simulink model "sdpm_vector_velocity"  (Simulink 9.0)
settings: Solver=ode45  StartTime=0.0  StopTime=5  RelTol=1e-7  AbsTol=1e-7  EnableMultiTasking=on
values from neighbouring files (symbols this model uses):
  c = 5    [index.m]
  iff = 10*0.71    (= 7.1)    [index.m]
  J = 0.00001    (= 1e-05)    [index.m]
  J2 = 0.000215    [index.m]
  ki1 = 20000    [index.m]
  kii = ki*ki/4    (= 109202500)    [index.m]
  km = 3*(Lm*iff*pn)/2    (= 0.19809)    [index.m]
  kw = 0.04    [index.m]
  L = 0.008    [index.m]
  Lm = 0.0062    [index.m]
  nu = 0.00007/2    (= 3.5e-05)    [index.m]
  nu2 = nu    (= 3.5e-05)    [index.m]
  nu3 = 0.01    [index.m]
  pn = 3    [index.m]
  R = 7.2    [index.m]
  tau = 1/wo    [index.m]
settings Model: Creator=Alex  LastModifiedBy=Alexander
settings DataIOCC: LimitDataPoints=on  SignalLoggingSaveFormat=ModelDataLogs
settings OptimizationCC: ExpressionDepthLimit=2147483647
settings DebuggingCC: SolverPrmCheckMsg=warning  FcnCallInpInsideContextMsg=warning  StateNameClashWarn=warning
settings GRTTargetCC: GeneratePreprocessorConditionals=Disable all  CombineOutputUpdateFcns=off  GRTInterface=on

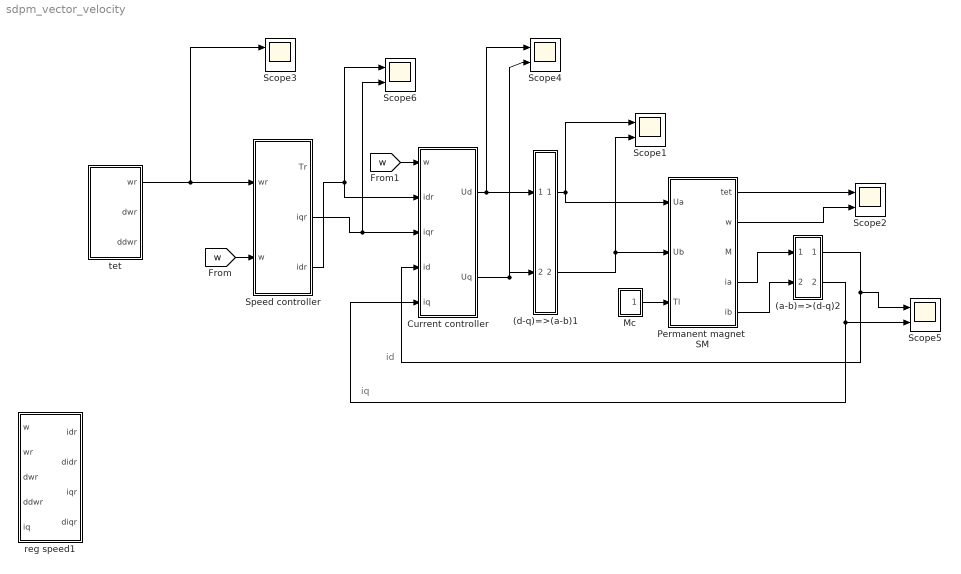
== system sdpm_vector_velocity ==
  note: id
  note: iq
  (a-b)=>(d-q)2 : Subsystem
  (d-q)=>(a-b)1 : Subsystem
  Current controller : Subsystem
  Mc : Subsystem  mask{te=1, td=1.5, Mc=0}
      mask prompts: te "Enable time"; td "Disable time"
  Permanent magnet  SM : Subsystem
  Scope{1..6} (6 alike) : Scope  NumInputPorts=2
  Speed controller : Subsystem
  reg speed1 : Subsystem  mask{kw=100, J=0.003, km=0.636, ktet=0}
      mask init:
      | kwi=(kw*kw)/2
  tet : Subsystem  mask{wrmax=1000, ta=0.5, ka=0.2, tcon=1, tex=0.5}
      mask prompts: wrmax "Final speed value"; ta "Ramp time"; ka "Coef. smooth"; tcon "Const speed time"; tex "Excitation time"
  wires:
  Mc/1(Mc) -> Permanent magnet  SM/3(Tl)
  tet/1(wr) -> Scope3/1, Speed controller/1(wr)
  Current controller/2(Uq) -> (d-q)=>(a-b)1/2("q "), Scope4/2
  (d-q)=>(a-b)1/2(b) -> Scope1/2, Permanent magnet  SM/2(Ub)
  (d-q)=>(a-b)1/1(a) -> Scope1/1, Permanent magnet  SM/1(Ua)
  (a-b)=>(d-q)2/2(q) -> Scope5/2, Current controller/5(iq)
  Speed controller/2("iqr  ") -> Scope6/2, Current controller/3(iqr)
  Current controller/1(Ud) -> Scope4/1, (d-q)=>(a-b)1/1(d)
  (a-b)=>(d-q)2/1(d) -> Scope5/1, Current controller/4(id)
  Speed controller/3(idr) -> Scope6/1, Current controller/2(idr)
  [w] -> Speed controller/2("w ")
  [w] -> Current controller/1(w)
  Permanent magnet  SM/1(tet) -> Scope2/1
  Permanent magnet  SM/2(w) -> Scope2/2
  Permanent magnet  SM/4(ia) -> (a-b)=>(d-q)2/1(a)
  Permanent magnet  SM/5(ib) -> (a-b)=>(d-q)2/2("b ")

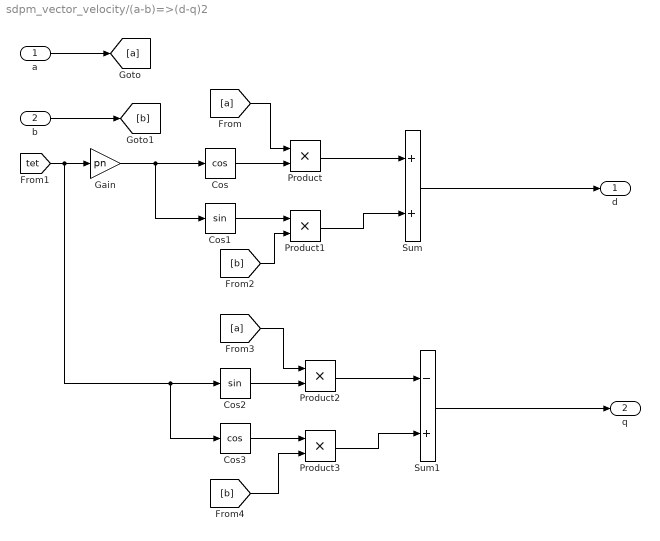
== system sdpm_vector_velocity/(a-b)=>(d-q)2 ==
  a : Inport
  "b " : Inport  Port=2
  Cos : Trigonometry  Operator=cos
  Cos1 : Trigonometry
  Cos2 : Trigonometry
  Cos3 : Trigonometry  Operator=cos
  Gain : Gain  Gain=pn
  Product{,1..3} (4 alike) : Product
  Sum : Sum
  Sum1 : Sum  Inputs=-+
  d : Outport
  q : Outport  Port=2
  wires:
  [b] -> Product1/2
  [b] -> Product3/2
  a/1 -> [a]
  [a] -> Product/1
  Sum/1 -> d/1
  [a] -> Product2/1
  Sum1/1 -> q/1
  Cos3/1 -> Product3/1
  Product3/1 -> Sum1/2
  Product/1 -> Sum/1
  Product2/1 -> Sum1/1
  Gain/1 -> Cos1/1, Cos/1
  Product1/1 -> Sum/2
  Cos1/1 -> Product1/1
  "b "/1 -> [b]
  Cos/1 -> Product/2
  [tet] -> Cos3/1, Cos2/1, Gain/1
  Cos2/1 -> Product2/2

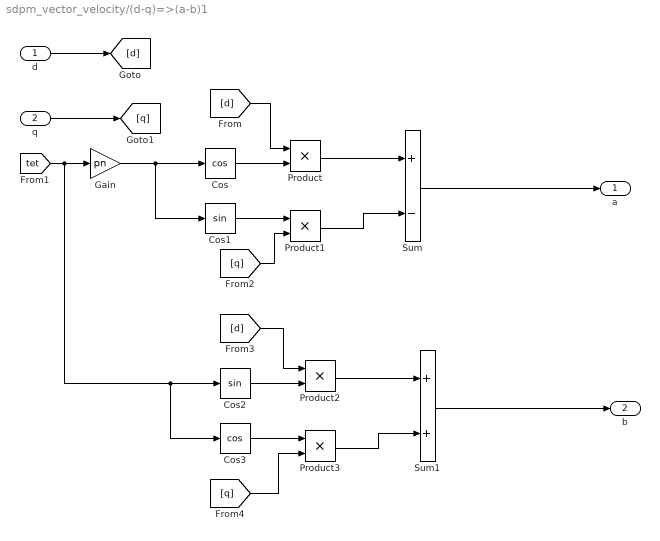
== system sdpm_vector_velocity/(d-q)=>(a-b)1 ==
  d : Inport
  "q " : Inport  Port=2
  Cos : Trigonometry  Operator=cos
  Cos1 : Trigonometry
  Cos2 : Trigonometry
  Cos3 : Trigonometry  Operator=cos
  Gain : Gain  Gain=pn
  Product{,1..3} (4 alike) : Product
  Sum : Sum  Inputs=+-
  Sum1 : Sum
  a : Outport
  b : Outport  Port=2
  wires:
  Gain/1 -> Cos1/1, Cos/1
  Cos/1 -> Product/2
  Product/1 -> Sum/1
  Cos1/1 -> Product1/1
  Product1/1 -> Sum/2
  Sum/1 -> a/1
  Product2/1 -> Sum1/1
  Cos2/1 -> Product2/2
  Sum1/1 -> b/1
  [tet] -> Cos3/1, Cos2/1, Gain/1
  Product3/1 -> Sum1/2
  Cos3/1 -> Product3/1
  d/1 -> [d]
  "q "/1 -> [q]
  [d] -> Product/1
  [q] -> Product1/2
  [d] -> Product2/1
  [q] -> Product3/2

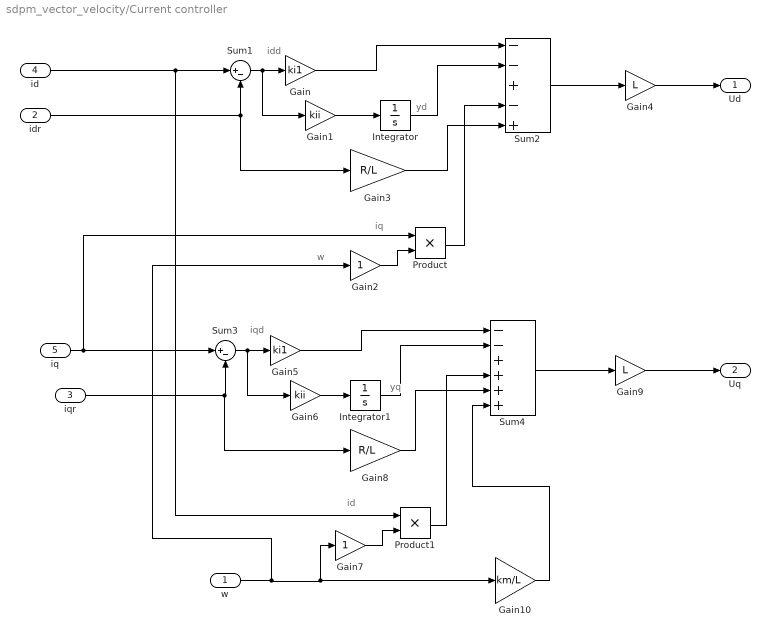
== system sdpm_vector_velocity/Current controller ==
  note: yq
  note: iqd
  note: yd
  note: idd
  note: w
  note: iq
  note: id
  w : Inport
  idr : Inport  Port=2
  iqr : Inport  Port=3
  id : Inport  Port=4
  iq : Inport  Port=5
  Gain : Gain  Gain=ki1
  Gain1 : Gain  Gain=kii
  Gain10 : Gain  Gain=km/L
  Gain2 : Gain
  Gain3 : Gain  Gain=R/L
  Gain4 : Gain  Gain=L
  Gain5 : Gain  Gain=ki1
  Gain6 : Gain  Gain=kii
  Gain7 : Gain
  Gain8 : Gain  Gain=R/L
  Gain9 : Gain  Gain=L
  Integrator : Integrator
  Integrator1 : Integrator
  Product : Product
  Product1 : Product
  Sum1 : Sum  Inputs=|+-
  Sum2 : Sum  Inputs=--+-+
  Sum3 : Sum  Inputs=|+-
  Sum4 : Sum  Inputs=--++++
  Ud : Outport
  Uq : Outport  Port=2
  wires:
  Product/1 -> Sum2/4
  Sum2/1 -> Gain4/1
  w/1 -> Gain7/1, Gain10/1, Gain2/1
  Integrator1/1 -> Sum4/2
  Gain7/1 -> Product1/2
  Gain8/1 -> Sum4/5
  Sum4/1 -> Gain9/1
  Gain9/1 -> Uq/1
  Product1/1 -> Sum4/4
  Gain6/1 -> Integrator1/1
  Sum3/1 -> Gain5/1, Gain6/1
  iqr/1 -> Sum3/2, Gain8/1
  Gain5/1 -> Sum4/1
  Gain4/1 -> Ud/1
  idr/1 -> Sum1/2, Gain3/1
  Sum1/1 -> Gain/1, Gain1/1
  id/1 -> Sum1/1, Product1/1
  iq/1 -> Product/1, Sum3/1
  Gain2/1 -> Product/2
  Gain/1 -> Sum2/1
  Gain10/1 -> Sum4/6
  Integrator/1 -> Sum2/2
  Gain3/1 -> Sum2/5
  Gain1/1 -> Integrator/1

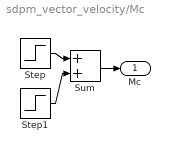
== system sdpm_vector_velocity/Mc ==
  Step : Step  Time=te  After=Mc
  Step1 : Step  Time=td  After=-Mc
  Sum : Sum  SaturateOnIntegerOverflow=on  InputSameDT=on  OutDataTypeStr=Inherit: Same as first input
  Mc : Outport
  wires:
  Step/1 -> Sum/1
  Step1/1 -> Sum/2
  Sum/1 -> Mc/1

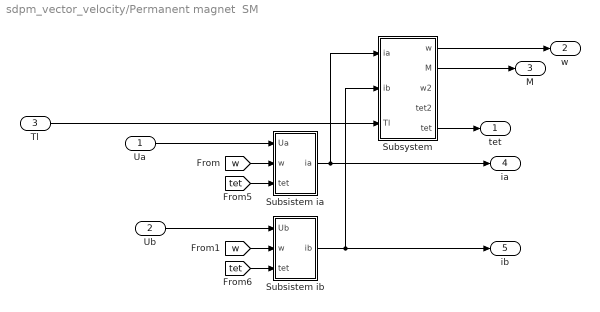
== system sdpm_vector_velocity/Permanent magnet  SM ==
  Ua : Inport
  Ub : Inport  Port=2
  Tl : Inport  Port=3
  Subsistem ia : Subsystem
  Subsistem ib : Subsystem
  Subsystem : Subsystem
  tet : Outport
  w : Outport  Port=2
  M : Outport  Port=3
  ia : Outport  Port=4
  ib : Outport  Port=5
  wires:
  Ua/1 -> Subsistem ia/1(Ua)
  Subsistem ia/1(ia) -> ia/1, Subsystem/1(ia)
  Ub/1 -> Subsistem ib/1(Ub)
  Subsistem ib/1(ib) -> ib/1, Subsystem/2(ib)
  Subsystem/2(M) -> M/1
  Tl/1 -> Subsystem/3("Tl ")
  Subsystem/1(w) -> w/1
  [w] -> Subsistem ia/2(w)
  [w] -> Subsistem ib/2(w)
  [tet] -> Subsistem ia/3(tet)
  [tet] -> Subsistem ib/3(tet)
  Subsystem/5(tet) -> tet/1

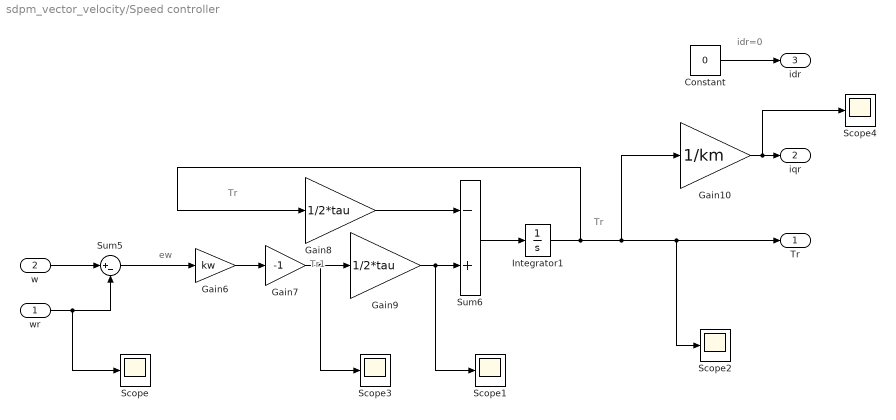
== system sdpm_vector_velocity/Speed controller ==
  note: idr=0
  note: Tr1
  note: ew
  note: Tr
  note: Tr
  wr : Inport
  "w " : Inport  Port=2
  Constant : Constant  Value=0
  Gain10 : Gain  Gain=1/km
  Gain6 : Gain  Gain=kw
  Gain7 : Gain  Gain=-1
  Gain8 : Gain  Gain=1/2*tau
  Gain9 : Gain  Gain=1/2*tau
  Integrator1 : Integrator
  Scope{,1..4} (5 alike) : Scope
  Sum5 : Sum  Inputs=|+-
  Sum6 : Sum  Inputs=-+
  Tr : Outport
  "iqr  " : Outport  Port=2
  idr : Outport  Port=3
  wires:
  wr/1 -> Scope/1, Sum5/2
  "w "/1 -> Sum5/1
  Sum5/1 -> Gain6/1
  Gain6/1 -> Gain7/1
  Gain7/1 -> Scope3/1, Gain9/1
  Integrator1/1 -> Gain8/1, Gain10/1, Scope2/1, Tr/1
  Sum6/1 -> Integrator1/1
  Gain9/1 -> Scope1/1, Sum6/2
  Gain8/1 -> Sum6/1
  Gain10/1 -> Scope4/1, "iqr  "/1
  Constant/1 -> idr/1

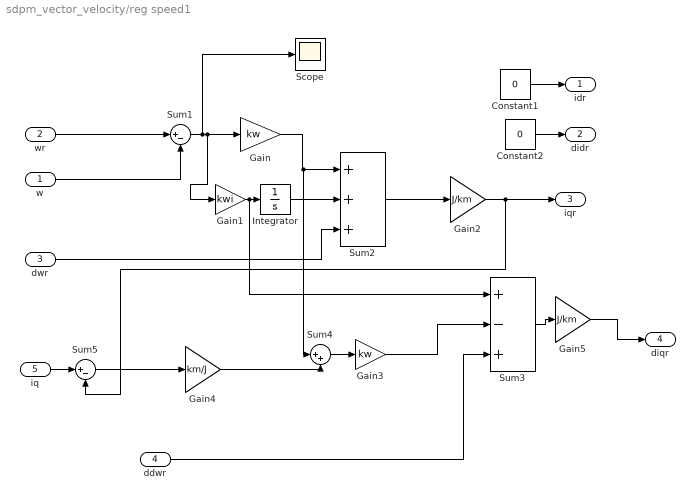
== system sdpm_vector_velocity/reg speed1 ==
  w : Inport
  wr : Inport  Port=2
  dwr : Inport  Port=3
  ddwr : Inport  Port=4
  iq : Inport  Port=5
  Constant1 : Constant  Value=0
  Constant2 : Constant  Value=0
  Gain : Gain  Gain=kw
  Gain1 : Gain  Gain=kwi
  Gain2 : Gain  Gain=J/km
  Gain3 : Gain  Gain=kw
  Gain4 : Gain  Gain=km/J
  Gain5 : Gain  Gain=J/km
  Integrator : Integrator
  Scope : Scope
  Sum1 : Sum  Inputs=|+-
  Sum2 : Sum  Inputs=+++
  Sum3 : Sum  Inputs=+-+
  Sum4 : Sum  Inputs=|++
  Sum5 : Sum  Inputs=|+-
  idr : Outport
  didr : Outport  Port=2
  iqr : Outport  Port=3
  diqr : Outport  Port=4
  wires:
  dwr/1 -> Sum2/3
  Gain5/1 -> diqr/1
  Sum3/1 -> Gain5/1
  ddwr/1 -> Sum3/3
  Gain3/1 -> Sum3/2
  Sum5/1 -> Gain4/1
  Gain4/1 -> Sum4/2
  Sum4/1 -> Gain3/1
  Integrator/1 -> Sum2/2
  Sum2/1 -> Gain2/1
  Gain2/1 -> iqr/1, Sum5/2
  w/1 -> Sum1/2
  wr/1 -> Sum1/1
  Gain1/1 -> Integrator/1, Sum3/1
  Sum1/1 -> Gain/1, Gain1/1, Scope/1
  Gain/1 -> Sum2/1, Sum4/1
  iq/1 -> Sum5/1
  Constant1/1 -> idr/1
  Constant2/1 -> didr/1

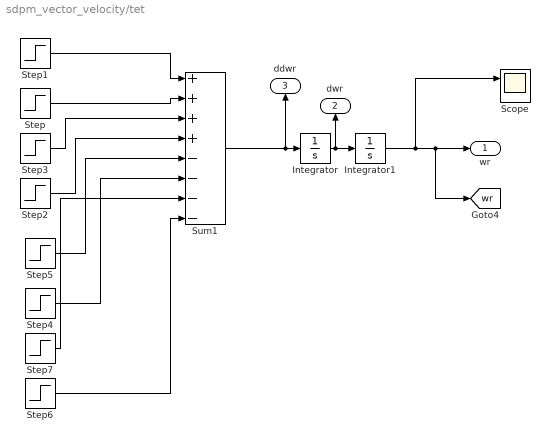
== system sdpm_vector_velocity/tet ==
  Integrator : Integrator
  Integrator1 : Integrator
  Scope : Scope  NumInputPorts=2
  Step : Step  Time=tex+ta*ka  After=-wrmax/(ka*ta*ka*ta+ka*ta*(ta-2*ka*ta))
  Step1 : Step  Time=tex  After=wrmax/(ka*ta*ka*ta+ka*ta*(ta-2*ka*ta))
  Step2 : Step  Time=tex+ta  After=wrmax/(ka*ta*ka*ta+ka*ta*(ta-2*ka*ta))
  Step3 : Step  Time=tex+ta*ka+(ta-2*ta*ka)  After=-wrmax/(ka*ta*ka*ta+ka*ta*(ta-2*ka*ta))
  Step4 : Step  Time=tex+ta+tcon+ta*ka  After=-wrmax/(ka*ta*ka*ta+ka*ta*(ta-2*ka*ta))
  Step5 : Step  Time=tex+ta+tcon  After=wrmax/(ka*ta*ka*ta+ka*ta*(ta-2*ka*ta))
  Step6 : Step  Time=tex+ta+tcon+ta  After=wrmax/(ka*ta*ka*ta+ka*ta*(ta-2*ka*ta))
  Step7 : Step  Time=tex+ta+tcon+ta*ka+(ta-2*ta*ka)  After=-wrmax/(ka*ta*ka*ta+ka*ta*(ta-2*ka*ta))
  Sum1 : Sum  Inputs=++++----  SaturateOnIntegerOverflow=on  InputSameDT=on  OutDataTypeStr=Inherit: Same as first input
  wr : Outport  InitialOutput=0
  dwr : Outport  Port=2  InitialOutput=0
  ddwr : Outport  Port=3  InitialOutput=0
  tag scope: wr=global
  wires:
  Step6/1 -> Sum1/8
  Step7/1 -> Sum1/7
  Step4/1 -> Sum1/6
  Integrator/1 -> dwr/1, Integrator1/1
  Sum1/1 -> Integrator/1, ddwr/1
  Integrator1/1 -> wr/1, [wr], Scope/1
  Step5/1 -> Sum1/5
  Step2/1 -> Sum1/4
  Step3/1 -> Sum1/3
  Step/1 -> Sum1/2
  Step1/1 -> Sum1/1

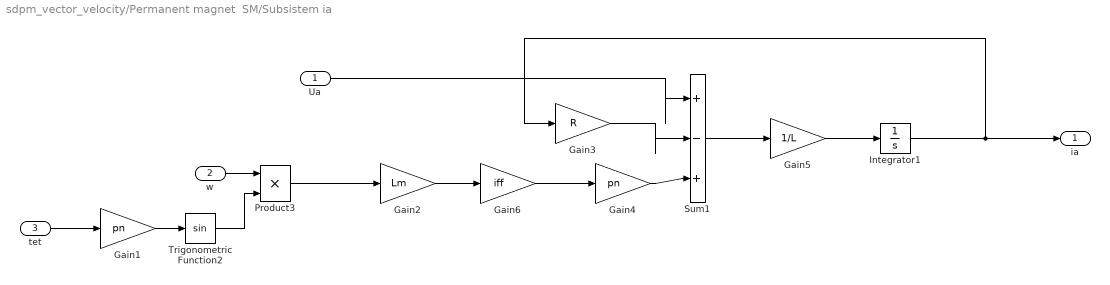
== system sdpm_vector_velocity/Permanent magnet  SM/Subsistem ia ==
  Ua : Inport
  w : Inport  Port=2
  tet : Inport  Port=3
  Gain1 : Gain  Gain=pn  SaturateOnIntegerOverflow=on  OutDataTypeStr=Inherit: Same as input  ParamDataTypeStr=Inherit: Same as input
  Gain2 : Gain  Gain=Lm  SaturateOnIntegerOverflow=on  OutDataTypeStr=Inherit: Same as input  ParamDataTypeStr=Inherit: Same as input
  Gain3 : Gain  Gain=R  SaturateOnIntegerOverflow=on  OutDataTypeStr=Inherit: Same as input  ParamDataTypeStr=Inherit: Same as input
  Gain4 : Gain  Gain=pn  SaturateOnIntegerOverflow=on  OutDataTypeStr=Inherit: Same as input  ParamDataTypeStr=Inherit: Same as input
  Gain5 : Gain  Gain=1/L  SaturateOnIntegerOverflow=on  OutDataTypeStr=Inherit: Same as input  ParamDataTypeStr=Inherit: Same as input
  Gain6 : Gain  Gain=iff  SaturateOnIntegerOverflow=on  OutDataTypeStr=Inherit: Same as input  ParamDataTypeStr=Inherit: Same as input
  Integrator1 : Integrator
  Product3 : Product  SaturateOnIntegerOverflow=on  RndMeth=Zero  InputSameDT=on  OutDataTypeStr=Inherit: Same as first input
  Sum1 : Sum  Inputs=|+-+
  Trigonometric Function2 : Trigonometry
  ia : Outport
  wires:
  Sum1/1 -> Gain5/1
  Gain4/1 -> Sum1/3
  Gain3/1 -> Sum1/2
  Ua/1 -> Sum1/1
  Product3/1 -> Gain2/1
  Trigonometric Function2/1 -> Product3/2
  Gain5/1 -> Integrator1/1
  Integrator1/1 -> ia/1, Gain3/1
  w/1 -> Product3/1
  Gain1/1 -> Trigonometric Function2/1
  tet/1 -> Gain1/1
  Gain2/1 -> Gain6/1
  Gain6/1 -> Gain4/1

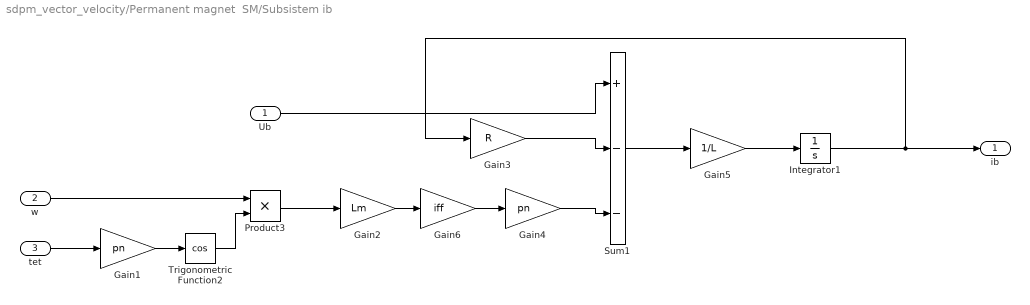
== system sdpm_vector_velocity/Permanent magnet  SM/Subsistem ib ==
  Ub : Inport
  w : Inport  Port=2
  tet : Inport  Port=3
  Gain1 : Gain  Gain=pn  SaturateOnIntegerOverflow=on  OutDataTypeStr=Inherit: Same as input  ParamDataTypeStr=Inherit: Same as input
  Gain2 : Gain  Gain=Lm  SaturateOnIntegerOverflow=on  OutDataTypeStr=Inherit: Same as input  ParamDataTypeStr=Inherit: Same as input
  Gain3 : Gain  Gain=R  SaturateOnIntegerOverflow=on  OutDataTypeStr=Inherit: Same as input  ParamDataTypeStr=Inherit: Same as input
  Gain4 : Gain  Gain=pn  SaturateOnIntegerOverflow=on  OutDataTypeStr=Inherit: Same as input  ParamDataTypeStr=Inherit: Same as input
  Gain5 : Gain  Gain=1/L  SaturateOnIntegerOverflow=on  OutDataTypeStr=Inherit: Same as input  ParamDataTypeStr=Inherit: Same as input
  Gain6 : Gain  Gain=iff  SaturateOnIntegerOverflow=on  OutDataTypeStr=Inherit: Same as input  ParamDataTypeStr=Inherit: Same as input
  Integrator1 : Integrator
  Product3 : Product  SaturateOnIntegerOverflow=on  RndMeth=Zero  InputSameDT=on  OutDataTypeStr=Inherit: Same as first input
  Sum1 : Sum  Inputs=|+--
  Trigonometric Function2 : Trigonometry  Operator=cos
  ib : Outport
  wires:
  Sum1/1 -> Gain5/1
  Gain4/1 -> Sum1/3
  Gain3/1 -> Sum1/2
  Ub/1 -> Sum1/1
  Trigonometric Function2/1 -> Product3/2
  Gain5/1 -> Integrator1/1
  Integrator1/1 -> ib/1, Gain3/1
  w/1 -> Product3/1
  Gain1/1 -> Trigonometric Function2/1
  tet/1 -> Gain1/1
  Gain2/1 -> Gain6/1
  Gain6/1 -> Gain4/1
  Product3/1 -> Gain2/1

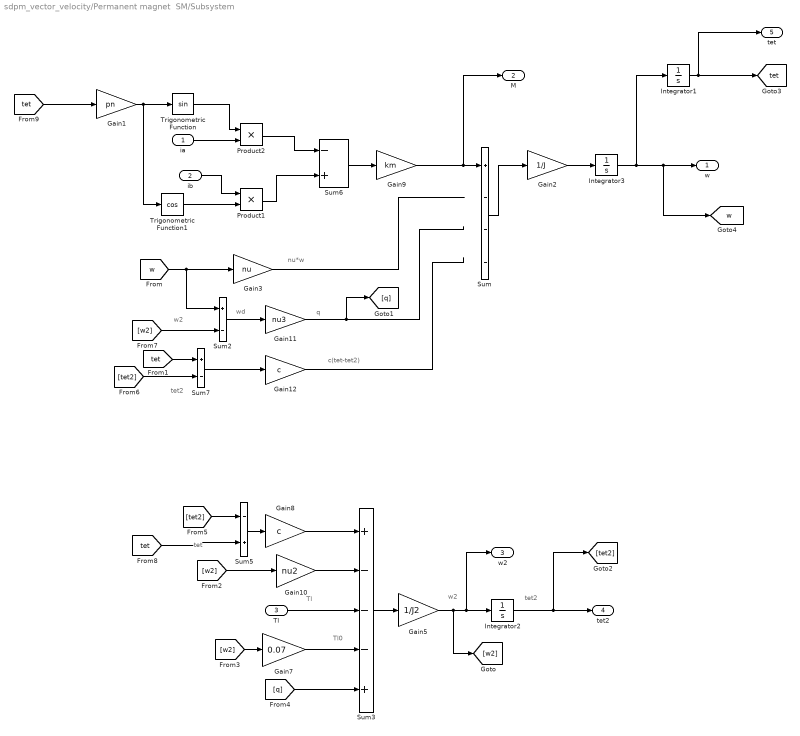
== system sdpm_vector_velocity/Permanent magnet  SM/Subsystem ==
  note: c(tet-tet2)
  note: tet2
  note: q
  note: wd
  note: w2
  note: nu*w
  note: w2
  note: tet2
  note: Tl0
  note: tet
  note: Tl
  ia : Inport
  ib : Inport  Port=2
  "Tl " : Inport  Port=3
  Gain1 : Gain  Gain=pn  SaturateOnIntegerOverflow=on  OutDataTypeStr=Inherit: Same as input  ParamDataTypeStr=Inherit: Same as input
  Gain10 : Gain  Gain=nu2  SaturateOnIntegerOverflow=on  OutDataTypeStr=Inherit: Same as input  ParamDataTypeStr=Inherit: Same as input
  Gain11 : Gain  Gain=nu3  SaturateOnIntegerOverflow=on  OutDataTypeStr=Inherit: Same as input  ParamDataTypeStr=Inherit: Same as input
  Gain12 : Gain  Gain=c  SaturateOnIntegerOverflow=on  OutDataTypeStr=Inherit: Same as input  ParamDataTypeStr=Inherit: Same as input
  Gain2 : Gain  Gain=1/J  SaturateOnIntegerOverflow=on  OutDataTypeStr=Inherit: Same as input  ParamDataTypeStr=Inherit: Same as input
  Gain3 : Gain  Gain=nu  SaturateOnIntegerOverflow=on  OutDataTypeStr=Inherit: Same as input  ParamDataTypeStr=Inherit: Same as input
  Gain5 : Gain  Gain=1/J2  SaturateOnIntegerOverflow=on  OutDataTypeStr=Inherit: Same as input  ParamDataTypeStr=Inherit: Same as input
  Gain7 : Gain  Gain=0.07  SaturateOnIntegerOverflow=on  OutDataTypeStr=Inherit: Same as input  ParamDataTypeStr=Inherit: Same as input
  Gain8 : Gain  Gain=c  SaturateOnIntegerOverflow=on  OutDataTypeStr=Inherit: Same as input  ParamDataTypeStr=Inherit: Same as input
  Gain9 : Gain  Gain=km  SaturateOnIntegerOverflow=on  OutDataTypeStr=Inherit: Same as input  ParamDataTypeStr=Inherit: Same as input
  Integrator1 : Integrator
  Integrator2 : Integrator
  Integrator3 : Integrator
  Product1 : Product  SaturateOnIntegerOverflow=on  RndMeth=Zero  InputSameDT=on  OutDataTypeStr=Inherit: Same as first input
  Product2 : Product  SaturateOnIntegerOverflow=on  RndMeth=Zero  InputSameDT=on  OutDataTypeStr=Inherit: Same as first input
  Sum : Sum  Inputs=+---
  Sum2 : Sum  Inputs=+-  SaturateOnIntegerOverflow=on  InputSameDT=on  OutDataTypeStr=Inherit: Same as first input
  Sum3 : Sum  Inputs=+---+  SaturateOnIntegerOverflow=on  InputSameDT=on  OutDataTypeStr=Inherit: Same as first input
  Sum5 : Sum  Inputs=-+  SaturateOnIntegerOverflow=on  InputSameDT=on  OutDataTypeStr=Inherit: Same as first input
  Sum6 : Sum  Inputs=-+  SaturateOnIntegerOverflow=on  InputSameDT=on  OutDataTypeStr=Inherit: Same as first input
  Sum7 : Sum  Inputs=+-  SaturateOnIntegerOverflow=on  InputSameDT=on  OutDataTypeStr=Inherit: Same as first input
  Trigonometric Function : Trigonometry
  Trigonometric Function1 : Trigonometry  Operator=cos
  w : Outport
  M : Outport  Port=2
  w2 : Outport  Port=3
  tet2 : Outport  Port=4
  tet : Outport  Port=5
  tag scope: tet=global, w=global
  wires:
  Gain9/1 -> M/1, Sum/1
  Integrator3/1 -> Integrator1/1, [w], w/1
  Sum/1 -> Gain2/1
  Product1/1 -> Sum6/2
  Trigonometric Function/1 -> Product2/1
  Sum6/1 -> Gain9/1
  Trigonometric Function1/1 -> Product1/2
  Product2/1 -> Sum6/1
  Gain2/1 -> Integrator3/1
  ia/1 -> Product2/2
  ib/1 -> Product1/1
  Gain1/1 -> Trigonometric Function/1, Trigonometric Function1/1
  [w] -> Sum2/1, Gain3/1
  Gain3/1 -> ?
  Sum5/1 -> Gain8/1
  Gain7/1 -> Sum3/4
  "Tl "/1 -> Sum3/3
  Gain10/1 -> Sum3/2
  Gain8/1 -> Sum3/1
  Sum3/1 -> Gain5/1
  Gain5/1 -> [w2], w2/1, Integrator2/1
  Integrator2/1 -> [tet2], tet2/1
  [w2] -> Sum2/2
  Sum2/1 -> Gain11/1
  Gain11/1 -> [q]
  [tet] -> Sum7/1
  [tet2] -> Sum7/2
  Sum7/1 -> Gain12/1
  Gain12/1 -> ?
  [w2] -> Gain10/1
  [w2] -> Gain7/1
  [q] -> Sum3/5
  [tet2] -> Sum5/1
  Integrator1/1 -> tet/1, [tet]
  [tet] -> Sum5/2
  [tet] -> Gain1/1
